simulink model "dlqrest_dist_3x3_2023"  (R2021b)
settings: Solver=ode23t  StartTime=0.0  StopTime=10.0  FixedStep=Ts/10  RelTol=1e-8  AbsTol=1e-9
values from neighbouring files (symbols this model uses):
  Bm = 2e-6    (= 2e-06)    [TEST_dist_effect_motor_2023.m]    (also in TestDIST_EFFECT_DCmotor.m = 1.5e-06)
  Festar1 = F1-L1*[1 0 0]    [TEST_dist_effect_motor_2023.m]    (also in TestDIST_EFFECT_DCmotor.m)
  Gestar1 = [G1 L1]    [TEST_dist_effect_motor_2023.m]    (also in TestDIST_EFFECT_DCmotor.m)
  Jt = Jm+J1+J2    (= 2.089856e-05)    [TEST_dist_effect_motor_2023.m]    (also in TestDIST_EFFECT_DCmotor.m)
  KK = dlqr(Fs,Gs,Q,R)    [TEST_dist_effect_motor_2023.m]    (also in TestDIST_EFFECT_DCmotor.m)
  Kt = 0.042    [TEST_dist_effect_motor_2023.m]    (also in TestDIST_EFFECT_DCmotor.m)
  Lm = 1.16e-3    (= 0.00116)    [TEST_dist_effect_motor_2023.m]    (also in TestDIST_EFFECT_DCmotor.m)
  Rm = 8.4    [TEST_dist_effect_motor_2023.m]    (also in TestDIST_EFFECT_DCmotor.m)
  Ts = 0.002    [TEST_dist_effect_motor_2023.m]    (also in TestDIST_EFFECT_DCmotor.m)
libraries: simulink x1
settings Model: Creator=oboe  LastModifiedBy=oboe
settings SolverCC: AutoScaleAbsTol=off  AlgebraicLoopSolver=TrustRegion
settings DataIOCC: ReturnWorkspaceOutputs=off
settings DebuggingCC: SFMachineParentedDataDiag=warning  ArithmeticOperatorsInVariantConditions=warning
settings SFSimCC: SimUseLocalCustomCode=off  CustomCodeUndefinedFunction=UseInterfaceOnly
settings RTWCC: RTWUseLocalCustomCode=off
settings CodeAppCC: StateflowObjectComments=on

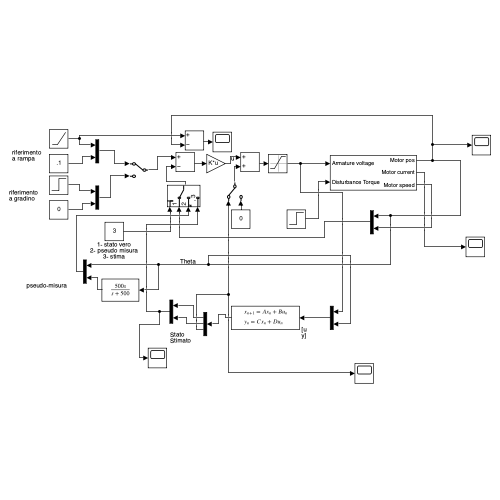
[thumbnail: Simulink's stored preview of the top-level diagram]
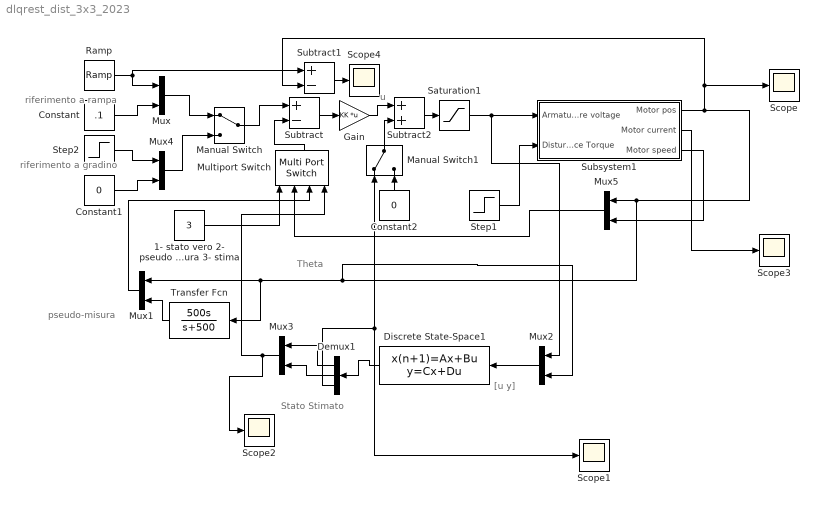
== system dlqrest_dist_3x3_2023 ==
  note: riferimento
      | a rampa
  note: pseudo-misura
  note: [u
      | y]
  note: Stato
      | Stimato
  note: u
  note: Theta
  note: riferimento
      | a gradino
  1- stato vero 2- pseudo misura 3- stima : Constant  Value=3
  Constant : Constant  Value=.1
  Constant1 : Constant  Value=0
  Constant2 : Constant  Value=0
  Demux1 : Demux  Outputs=3
  Discrete State-Space1 : DiscreteStateSpace  A=Festar1  B=Gestar1  C=eye(3)  D=[0 0; 0 0 ; 0 0]  InitialCondition=[0 0 0]'  SampleTime=Ts
  Gain : Gain  Gain=KK  Multiplication=Matrix(K*u)
  Manual Switch : ManualSwitch
  Manual Switch1 : ManualSwitch
  Multiport Switch : MultiPortSwitch
  Mux{,1..5} (6 alike) : Mux  Inputs=2
  Ramp : simulink/Sources/Ramp  slope=.1  start=0  InitialOutput=0
  Saturation1 : Saturate  UpperLimit=12  LowerLimit=-12
  Scope{,1..4} (5 alike) : Scope
  Step1 : Step  Time=3  After=0.01  SampleTime=0
  Step2 : Step  SampleTime=0
  Subsystem1 : Subsystem
  Subtract : Sum  Inputs=+-
  Subtract1 : Sum  Inputs=+-
  Subtract2 : Sum
  Transfer Fcn : TransferFcn  Numerator=[500 0]  Denominator=[1 500]
  wires:
  Subsystem1/1(Motor pos) -> Mux2/2, Transfer Fcn/1, Mux1/1, Mux5/1, Subtract1/2, Scope/1
  Subtract/1 -> Gain/1
  Constant/1 -> Mux/2
  Ramp/1 -> Subtract1/1, Mux/1
  Transfer Fcn/1 -> Mux1/2
  Mux2/1 -> Discrete State-Space1/1
  Mux1/1 -> Multiport Switch/3
  1- stato vero 2- pseudo misura 3- stima/1 -> Multiport Switch/1
  Multiport Switch/1 -> Subtract/2
  Saturation1/1 -> Subsystem1/1(Armature voltage), Mux2/1
  Step1/1 -> Subsystem1/2(Disturbance Torque)
  Subtract2/1 -> Saturation1/1
  Gain/1 -> Subtract2/1
  Demux1/1 -> Mux3/1
  Mux3/1 -> Scope2/1, Multiport Switch/4
  Discrete State-Space1/1 -> Demux1/1
  Constant1/1 -> Mux4/2
  Step2/1 -> Mux4/1
  Manual Switch/1 -> Subtract/1
  Mux/1 -> Manual Switch/1
  Mux4/1 -> Manual Switch/2
  Demux1/2 -> Mux3/2
  Demux1/3 -> Scope1/1, Manual Switch1/1
  Subsystem1/3(Motor speed) -> Mux5/2
  Mux5/1 -> Multiport Switch/2
  Manual Switch1/1 -> Subtract2/2
  Constant2/1 -> Manual Switch1/2
  Subsystem1/2(Motor current) -> Scope3/1
  Subtract1/1 -> Scope4/1

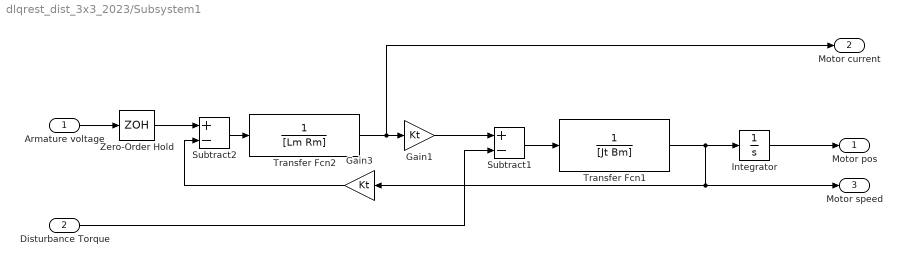
== system dlqrest_dist_3x3_2023/Subsystem1 ==
  Armature voltage : Inport
  Disturbance Torque : Inport  Port=2
  Gain1 : Gain  Gain=Kt
  Gain3 : Gain  Gain=Kt
  Integrator : Integrator
  Subtract1 : Sum  Inputs=+-
  Subtract2 : Sum  Inputs=+-
  Transfer Fcn1 : TransferFcn  Denominator=[Jt Bm]
  Transfer Fcn2 : TransferFcn  Denominator=[Lm Rm]
  Zero-Order Hold : ZeroOrderHold  SampleTime=.001
  Motor pos : Outport
  Motor current : Outport  Port=2
  Motor speed : Outport  Port=3
  wires:
  Integrator/1 -> Motor pos/1
  Zero-Order Hold/1 -> Subtract2/1
  Transfer Fcn2/1 -> Motor current/1, Gain1/1
  Gain3/1 -> Subtract2/2
  Subtract2/1 -> Transfer Fcn2/1
  Armature voltage/1 -> Zero-Order Hold/1
  Transfer Fcn1/1 -> Integrator/1, Gain3/1, Motor speed/1
  Subtract1/1 -> Transfer Fcn1/1
  Gain1/1 -> Subtract1/1
  Disturbance Torque/1 -> Subtract1/2
